simulink model "EiTR2018B (1)"  (R2019b)
settings: Solver=VariableStepAuto  StartTime=0.0  StopTime=600  RelTol=1e-3
values from neighbouring files (symbols this model uses):
  boardingTime = 15    [configFile.m]
  transportTime = 60    [configFile.m]
undefined symbols (not defined in the file or in its folder): m, n
(part 1 of 2)
settings Model: OrderedModelArguments=off  Creator=haavi  LastModifiedBy=eivin
settings DebuggingCC: ArithmeticOperatorsInVariantConditions=warning
settings SFSimCC: CustomCodeUndefinedFunction=UseInterfaceOnly

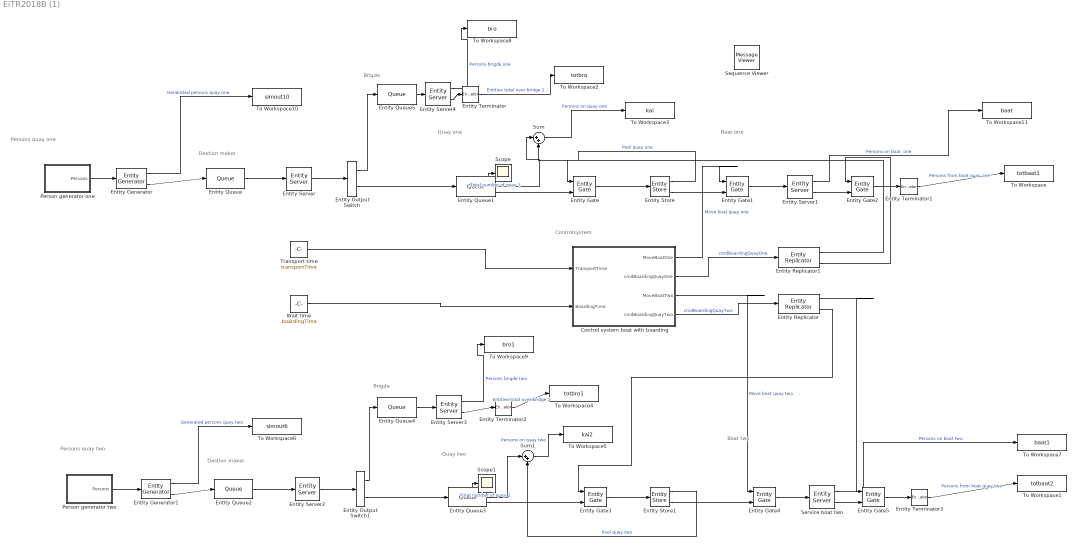
== system EiTR2018B (1) ==
  note: Controlsystem
  note: Persons quay two
  note: Boat one
  note: Quay one
  note: Brigde
  note: Destion maker
  note: Persons quay one
  note: Destion maker
  note: Brigde
  note: Quay two
  note: Boat two
  Control system boat with boarding : Stateflow chart  TreatAsAtomicUnit=on
  Entity Output Switch : EntityOutputSwitch  InputPortMessageModes=m  OutputPortMessageModes=m,m  SwitchingCriterion=From attribute  SwitchAttributeName=route
  Entity Output Switch1 : EntityOutputSwitch  InputPortMessageModes=m  OutputPortMessageModes=m,m  SwitchingCriterion=From attribute  SwitchAttributeName=route
  Entity Gate{,1..5} (6 alike) : EntityGate  InputPortMessageModes=m,m  OutputPortMessageModes=m
  Entity Generator : EntityGenerator  InputPortMessageModes=m  OutputPortMessageModes=n,m  GenerationMethod=Event-based  AttributeName=destion|route  AttributeInitialValue=-1|-1  NumberEntitiesDeparted=on  EntityType=Structured  EntityTypeName=person
      settings: InputPortMap=u0  OutputPortMap=o0,o3
  Entity Generator1 : EntityGenerator  InputPortMessageModes=m  OutputPortMessageModes=n,m  GenerationMethod=Event-based  AttributeName=destion|route  AttributeInitialValue=-1|-1  NumberEntitiesDeparted=on  EntityType=Structured  EntityTypeName=person2
      settings: InputPortMap=u0  OutputPortMap=o0,o3
  Entity Queue{,2,4..5} (4 alike) : Queue  InputPortMessageModes=m  OutputPortMessageModes=m  Capacity=inf
  Entity Queue1 : Queue  InputPortMessageModes=m  OutputPortMessageModes=n,n,m  Capacity=inf  NumberEntitiesDeparted=on  NumberEntitiesInBlock=on
      settings: OutputPortMap=o0,o1,o5
  Entity Queue3 : Queue  InputPortMessageModes=m  OutputPortMessageModes=n,n,m  Capacity=inf  NumberEntitiesDeparted=on  NumberEntitiesInBlock=on
      settings: OutputPortMap=o0,o1,o5
  Entity Replicator : EntityReplicator  InputPortMessageModes=m  OutputPortMessageModes=m,m
  Entity Replicator1 : EntityReplicator  InputPortMessageModes=m  OutputPortMessageModes=m,m
  Entity Server : EntityServer  InputPortMessageModes=m  OutputPortMessageModes=m  Capacity=inf  ServiceTimeValue=0  EntryAction=|
      | destion = 0.659;
      | entity.destion = rand();
      | 
      | if entity.destion >= destion
      |     entity.route = 1;
      | else
      |     entity.route = 2;
      | end
  Entity Server1 : EntityServer  InputPortMessageModes=m  OutputPortMessageModes=n,m  Capacity=maxPersonBoat  ServiceTimeValue=transportTime  NumberEntitiesInBlock=on
      settings: OutputPortMap=o1,o9
  Entity Server2 : EntityServer  InputPortMessageModes=m  OutputPortMessageModes=m  Capacity=inf  ServiceTimeValue=0  EntryAction=|
      | destion = 0.659;
      | entity.destion = rand();
      | 
      | if entity.destion >= destion
      |     entity.route = 1;
      | else
      |     entity.route = 2;
      | end
  Entity Server3 : EntityServer  InputPortMessageModes=m  OutputPortMessageModes=n,m  Capacity=inf  ServiceTimeValue=transportTimeBrigde  NumberEntitiesInBlock=on
      settings: OutputPortMap=o1,o9
  Entity Server4 : EntityServer  InputPortMessageModes=m  OutputPortMessageModes=n,m  Capacity=inf  ServiceTimeValue=transportTimeBrigde  NumberEntitiesInBlock=on
      settings: OutputPortMap=o1,o9
  Entity Store : EntityStore  InputPortMessageModes=m  OutputPortMessageModes=n,m  Capacity=maxPersonBoat  NumberEntitiesInBlock=on
      settings: OutputPortMap=o1,o4
  Entity Store1 : EntityStore  InputPortMessageModes=m  OutputPortMessageModes=n,m  Capacity=maxPersonBoat  NumberEntitiesInBlock=on
      settings: OutputPortMap=o1,o4
  Entity Terminator{,1..3} (4 alike) : EntityTerminator  InputPortMessageModes=m  NumberEntitiesArrived=on
      settings: OutputPortMap=o0
  Person generator one : Stateflow chart  TreatAsAtomicUnit=on
  Person generator two : Stateflow chart  TreatAsAtomicUnit=on
  Scope : Scope
  Scope1 : Scope
  Sequence Viewer : MessageViewer
  Service boat two : EntityServer  InputPortMessageModes=m  OutputPortMessageModes=n,m  Capacity=maxPersonBoat  ServiceTimeValue=transportTime  NumberEntitiesInBlock=on
      settings: OutputPortMap=o1,o9
  Sum : Sum  Inputs=|++
  Sum1 : Sum  Inputs=|++
  To Workspace : ToWorkspace  VariableName=totbaat1  SaveFormat=Timeseries  SampleTime=-1
  To Workspace1 : ToWorkspace  VariableName=totbaat2  SaveFormat=Timeseries  SampleTime=-1
  To Workspace10 : ToWorkspace  VariableName=simout10  SaveFormat=Timeseries  SampleTime=-1
  To Workspace11 : ToWorkspace  VariableName=baat  SaveFormat=Timeseries  SampleTime=-1
  To Workspace2 : ToWorkspace  VariableName=totbro  SaveFormat=Timeseries  SampleTime=-1
  To Workspace3 : ToWorkspace  VariableName=kai  SaveFormat=Timeseries  SampleTime=-1
  To Workspace4 : ToWorkspace  VariableName=totbro1  SaveFormat=Timeseries  SampleTime=-1
  To Workspace5 : ToWorkspace  VariableName=kai2  SaveFormat=Timeseries  SampleTime=-1
  To Workspace6 : ToWorkspace  VariableName=simout6  SaveFormat=Timeseries  SampleTime=-1
  To Workspace7 : ToWorkspace  VariableName=baat1  SaveFormat=Timeseries  SampleTime=-1
  To Workspace8 : ToWorkspace  VariableName=bro  SaveFormat=Timeseries  SampleTime=-1
  To Workspace9 : ToWorkspace  VariableName=bro1  SaveFormat=Timeseries  SampleTime=-1
  Transport time : Constant  Value=transportTime
  Wait time : Constant  Value=boardingTime
  wires:
  Entity Generator/2 -> Entity Queue/1
  Entity Queue/1 -> Entity Server/1
  Entity Server/1 -> Entity Output Switch/1
  Entity Output Switch/2 -> Entity Queue1/1
  Entity Generator1/2 -> Entity Queue2/1
  Entity Queue2/1 -> Entity Server2/1
  Entity Server2/1 -> Entity Output Switch1/1
  Entity Output Switch1/2 -> Entity Queue3/1
  Entity Queue3/3 -> Entity Gate3/2
  Entity Terminator1/1 -> To Workspace/1  "Persons from boat quay one"
  Entity Terminator3/1 -> To Workspace1/1  "Persons from boat quay two"
  Entity Terminator/1 -> To Workspace2/1  "Entities total over bridge 1"
  Entity Terminator2/1 -> To Workspace4/1  "Entities total over bridge 2"
  Person generator one/1(Persons) -> Entity Generator/1
  Person generator two/1(Persons) -> Entity Generator1/1
  Transport time/1 -> Control system boat with boarding/1(TransportTime)
  Wait time/1 -> Control system boat with boarding/2(BoardingTime)
  Service boat two/1 -> To Workspace7/1  "Persons on boat two"
  Entity Generator/1 -> To Workspace10/1  "Generated persons quay one"
  Entity Generator1/1 -> To Workspace6/1  "Generated persons quay two"
  Entity Queue1/3 -> Entity Gate/2
  Entity Gate/1 -> Entity Store/1
  Entity Store/2 -> Entity Gate1/2
  Control system boat with boarding/1(MoveBoatOne) -> Entity Gate1/1  "Move boat quay one"
  Entity Server1/1 -> To Workspace11/1  "Persons on boat  one"
  Entity Store/1 -> Sum/2  "Pool quay one"
  Entity Gate1/1 -> Entity Server1/1
  Entity Server1/2 -> Entity Gate2/2
  Entity Gate2/1 -> Entity Terminator1/1
  Control system boat with boarding/2(cmdBoardingQuayOne) -> Entity Replicator1/1  "cmdBoardingQuayOne"
  Entity Replicator1/1 -> Entity Gate/1
  Entity Replicator1/2 -> Entity Gate2/1
  Entity Queue1/2 -> Sum/1
  Sum/1 -> To Workspace3/1  "Persons on quay one"
  Control system boat with boarding/4(cmdBoardingQuayTwo) -> Entity Replicator/1  "cmdBoardingQuayTwo"
  Entity Gate3/1 -> Entity Store1/1
  Entity Store1/2 -> Entity Gate4/2
  Entity Gate4/1 -> Service boat two/1
  Entity Gate5/1 -> Entity Terminator3/1
  Service boat two/2 -> Entity Gate5/2
  Entity Replicator/1 -> Entity Gate5/1
  Entity Replicator/2 -> Entity Gate3/1
  Control system boat with boarding/3(MoveBoatTwo) -> Entity Gate4/1  "Move boat quay two"
  Entity Queue3/2 -> Sum1/1
  Entity Store1/1 -> Sum1/2  "Pool quay two"
  Sum1/1 -> To Workspace5/1  "Persons on quay two"
  Entity Server3/2 -> Entity Terminator2/1
  Entity Queue4/1 -> Entity Server3/1
  Entity Output Switch1/1 -> Entity Queue4/1
  Entity Output Switch/1 -> Entity Queue5/1
  Entity Queue5/1 -> Entity Server4/1
  Entity Server4/2 -> Entity Terminator/1
  Entity Server4/1 -> To Workspace8/1  "Persons brigde one"
  Entity Server3/1 -> To Workspace9/1  "Persons brigde two"
  Entity Queue1/1 -> Scope/1  "Total number of quay 1"
  Entity Queue3/1 -> Scope1/1  "Total number of quay 2"

== stateflow chart EiTR2018B (1)/Person generator one ==
  settings: enableNonTerminalStates=1
  state Hour_24
    state min_0
      state IDLE
        entry:
        lambda = 4;
        dt =60* rand();
        Persons.data=poissrnd(lambda);
      state Wait
      (default) -> Hour_24.min_0.IDLE
      Hour_24.min_0.Wait -> Hour_24.min_0.IDLE : after(dt,sec){send(Persons)}
      Hour_24.min_0.IDLE -> Hour_24.min_0.Wait
    state min_45
      state IDLE
        entry:
        lambda = 4;
        dt =60* rand();
        Persons.data=poissrnd(lambda);
      state Wait
      (default) -> Hour_24.min_45.IDLE : {dt=0;}
      Hour_24.min_45.Wait -> Hour_24.min_45.IDLE : after(dt,sec){send(Persons)}
      Hour_24.min_45.IDLE -> Hour_24.min_45.Wait
    state min_15
      state IDLE
        entry:
        lambda = 4;
        dt =60* rand();
        Persons.data=poissrnd(lambda);
      state Wait
      (default) -> Hour_24.min_15.IDLE : {dt=0;}
      Hour_24.min_15.Wait -> Hour_24.min_15.IDLE : after(dt,sec){send(Persons)}
      Hour_24.min_15.IDLE -> Hour_24.min_15.Wait
    state min_30
      state IDLE
        entry:
        lambda = 4;
        dt =60* rand();
        Persons.data=poissrnd(lambda);
      state Wait
      (default) -> Hour_24.min_30.IDLE : {dt=0;}
      Hour_24.min_30.Wait -> Hour_24.min_30.IDLE : after(dt,sec){send(Persons)}
      Hour_24.min_30.IDLE -> Hour_24.min_30.Wait
    (default) -> Hour_24.min_0
    Hour_24.min_0 -> Hour_24.min_15 : after(60*15,sec)
    Hour_24.min_30 -> Hour_24.min_45 : after(60*15,sec)
    Hour_24.min_15 -> Hour_24.min_30 : after(60*15,sec)
  state Hour_23
    state min_0
      state IDLE
        entry:
        lambda = 4;
        dt =60* rand();
        Persons.data=poissrnd(lambda);
      state Wait
      (default) -> Hour_23.min_0.IDLE
      Hour_23.min_0.Wait -> Hour_23.min_0.IDLE : after(dt,sec){send(Persons)}
      Hour_23.min_0.IDLE -> Hour_23.min_0.Wait
    state min_45
      state IDLE
        entry:
        lambda = 4;
        dt =60* rand();
        Persons.data=poissrnd(lambda);
      state Wait
      (default) -> Hour_23.min_45.IDLE : {dt=0;}
      Hour_23.min_45.Wait -> Hour_23.min_45.IDLE : after(dt,sec){send(Persons)}
      Hour_23.min_45.IDLE -> Hour_23.min_45.Wait
    state min_15
      state IDLE
        entry:
        lambda = 4;
        dt =60* rand();
        Persons.data=poissrnd(lambda);
      state Wait
      (default) -> Hour_23.min_15.IDLE : {dt=0;}
      Hour_23.min_15.Wait -> Hour_23.min_15.IDLE : after(dt,sec){send(Persons)}
      Hour_23.min_15.IDLE -> Hour_23.min_15.Wait
    state min_30
      state IDLE
        entry:
        lambda = 4;
        dt =60* rand();
        Persons.data=poissrnd(lambda);
      state Wait
      (default) -> Hour_23.min_30.IDLE : {dt=0;}
      Hour_23.min_30.Wait -> Hour_23.min_30.IDLE : after(dt,sec){send(Persons)}
      Hour_23.min_30.IDLE -> Hour_23.min_30.Wait
    (default) -> Hour_23.min_0
    Hour_23.min_0 -> Hour_23.min_15 : after(60*15,sec)
    Hour_23.min_30 -> Hour_23.min_45 : after(60*15,sec)
    Hour_23.min_15 -> Hour_23.min_30 : after(60*15,sec)
  state Hour_1
    state min_0
      state IDLE
        entry:
        lambda = 5;
        dt =60* rand()/poissrnd(lambda);
        Persons.data=poissrnd(lambda);
      state Wait
      (default) -> Hour_1.min_0.IDLE
      Hour_1.min_0.Wait -> Hour_1.min_0.IDLE : after(dt,sec){send(Persons)}
      Hour_1.min_0.IDLE -> Hour_1.min_0.Wait
    state min_45
      state IDLE
        entry:
        lambda = 4;
        dt =60* rand();
        Persons.data=poissrnd(lambda);
      state Wait
      (default) -> Hour_1.min_45.IDLE : {dt=0;}
      Hour_1.min_45.Wait -> Hour_1.min_45.IDLE : after(dt,sec){send(Persons)}
      Hour_1.min_45.IDLE -> Hour_1.min_45.Wait
    state min_15
      state IDLE
        entry:
        lambda = 40;
        dt =60* rand();
        Persons.data=poissrnd(lambda);
      state Wait
      (default) -> Hour_1.min_15.IDLE : {dt=0;}
      Hour_1.min_15.Wait -> Hour_1.min_15.IDLE : after(dt,sec){send(Persons)}
      Hour_1.min_15.IDLE -> Hour_1.min_15.Wait
    state min_30
      state IDLE
        entry:
        lambda = 4;
        dt =60* rand();
        Persons.data=poissrnd(lambda);
      state Wait
      (default) -> Hour_1.min_30.IDLE : {dt=0;}
      Hour_1.min_30.Wait -> Hour_1.min_30.IDLE : after(dt,sec){send(Persons)}
      Hour_1.min_30.IDLE -> Hour_1.min_30.Wait
    (default) -> Hour_1.min_0
    Hour_1.min_0 -> Hour_1.min_15 : after(60*15,sec)
    Hour_1.min_30 -> Hour_1.min_45 : after(60*15,sec)
    Hour_1.min_15 -> Hour_1.min_30 : after(60*15,sec)
  state Hour_22
    state min_0
      state IDLE
        entry:
        lambda = 4;
        dt =60* rand();
        Persons.data=poissrnd(lambda);
      state Wait
      (default) -> Hour_22.min_0.IDLE
      Hour_22.min_0.Wait -> Hour_22.min_0.IDLE : after(dt,sec){send(Persons)}
      Hour_22.min_0.IDLE -> Hour_22.min_0.Wait
    state min_45
      state IDLE
        entry:
        lambda = 4;
        dt =60* rand();
        Persons.data=poissrnd(lambda);
      state Wait
      (default) -> Hour_22.min_45.IDLE : {dt=0;}
      Hour_22.min_45.Wait -> Hour_22.min_45.IDLE : after(dt,sec){send(Persons)}
      Hour_22.min_45.IDLE -> Hour_22.min_45.Wait
    state min_15
      state IDLE
        entry:
        lambda = 4;
        dt =60* rand();
        Persons.data=poissrnd(lambda);
      state Wait
      (default) -> Hour_22.min_15.IDLE : {dt=0;}
      Hour_22.min_15.Wait -> Hour_22.min_15.IDLE : after(dt,sec){send(Persons)}
      Hour_22.min_15.IDLE -> Hour_22.min_15.Wait
    state min_30
      state IDLE
        entry:
        lambda = 4;
        dt =60* rand();
        Persons.data=poissrnd(lambda);
      state Wait
      (default) -> Hour_22.min_30.IDLE : {dt=0;}
      Hour_22.min_30.Wait -> Hour_22.min_30.IDLE : after(dt,sec){send(Persons)}
      Hour_22.min_30.IDLE -> Hour_22.min_30.Wait
    (default) -> Hour_22.min_0
    Hour_22.min_0 -> Hour_22.min_15 : after(60*15,sec)
    Hour_22.min_30 -> Hour_22.min_45 : after(60*15,sec)
    Hour_22.min_15 -> Hour_22.min_30 : after(60*15,sec)
  state Hour_2
    state min_0
      state IDLE
        entry:
        lambda = 4;
        dt =60* rand();
        Persons.data=poissrnd(lambda);
      state Wait
      (default) -> Hour_2.min_0.IDLE
      Hour_2.min_0.Wait -> Hour_2.min_0.IDLE : after(dt,sec){send(Persons)}
      Hour_2.min_0.IDLE -> Hour_2.min_0.Wait
    state min_45
      state IDLE
        entry:
        lambda = 4;
        dt =60* rand();
        Persons.data=poissrnd(lambda);
      state Wait
      (default) -> Hour_2.min_45.IDLE : {dt=0;}
      Hour_2.min_45.Wait -> Hour_2.min_45.IDLE : after(dt,sec){send(Persons)}
      Hour_2.min_45.IDLE -> Hour_2.min_45.Wait
    state min_15
      state IDLE
        entry:
        lambda = 4;
        dt =60* rand();
        Persons.data=poissrnd(lambda);
      state Wait
      (default) -> Hour_2.min_15.IDLE : {dt=0;}
      Hour_2.min_15.Wait -> Hour_2.min_15.IDLE : after(dt,sec){send(Persons)}
      Hour_2.min_15.IDLE -> Hour_2.min_15.Wait
    state min_30
      state IDLE
        entry:
        lambda = 4;
        dt =60* rand();
        Persons.data=poissrnd(lambda);
      state Wait
      (default) -> Hour_2.min_30.IDLE : {dt=0;}
      Hour_2.min_30.Wait -> Hour_2.min_30.IDLE : after(dt,sec){send(Persons)}
      Hour_2.min_30.IDLE -> Hour_2.min_30.Wait
    (default) -> Hour_2.min_0
    Hour_2.min_0 -> Hour_2.min_15 : after(60*15,sec)
    Hour_2.min_30 -> Hour_2.min_45 : after(60*15,sec)
    Hour_2.min_15 -> Hour_2.min_30 : after(60*15,sec)
  state Hour_21
    state min_0
      state IDLE
        entry:
        lambda = 4;
        dt =60* rand();
        Persons.data=poissrnd(lambda);
      state Wait
      (default) -> Hour_21.min_0.IDLE
      Hour_21.min_0.Wait -> Hour_21.min_0.IDLE : after(dt,sec){send(Persons)}
      Hour_21.min_0.IDLE -> Hour_21.min_0.Wait
    state min_45
      state IDLE
        entry:
        lambda = 4;
        dt =60* rand();
        Persons.data=poissrnd(lambda);
      state Wait
      (default) -> Hour_21.min_45.IDLE : {dt=0;}
      Hour_21.min_45.Wait -> Hour_21.min_45.IDLE : after(dt,sec){send(Persons)}
      Hour_21.min_45.IDLE -> Hour_21.min_45.Wait
    state min_15
      state IDLE
        entry:
        lambda = 4;
        dt =60* rand();
        Persons.data=poissrnd(lambda);
      state Wait
      (default) -> Hour_21.min_15.IDLE : {dt=0;}
      Hour_21.min_15.Wait -> Hour_21.min_15.IDLE : after(dt,sec){send(Persons)}
      Hour_21.min_15.IDLE -> Hour_21.min_15.Wait
    state min_30
      state IDLE
        entry:
        lambda = 4;
        dt =60* rand();
        Persons.data=poissrnd(lambda);
      state Wait
      (default) -> Hour_21.min_30.IDLE : {dt=0;}
      Hour_21.min_30.Wait -> Hour_21.min_30.IDLE : after(dt,sec){send(Persons)}
      Hour_21.min_30.IDLE -> Hour_21.min_30.Wait
    (default) -> Hour_21.min_0
    Hour_21.min_0 -> Hour_21.min_15 : after(60*15,sec)
    Hour_21.min_30 -> Hour_21.min_45 : after(60*15,sec)
    Hour_21.min_15 -> Hour_21.min_30 : after(60*15,sec)
  state Hour_3
    state min_0
      state IDLE
        entry:
        lambda = 4;
        dt =60* rand();
        Persons.data=poissrnd(lambda);
      state Wait
      (default) -> Hour_3.min_0.IDLE
      Hour_3.min_0.Wait -> Hour_3.min_0.IDLE : after(dt,sec){send(Persons)}
      Hour_3.min_0.IDLE -> Hour_3.min_0.Wait
    state min_45
      state IDLE
        entry:
        lambda = 4;
        dt =60* rand();
        Persons.data=poissrnd(lambda);
      state Wait
      (default) -> Hour_3.min_45.IDLE : {dt=0;}
      Hour_3.min_45.Wait -> Hour_3.min_45.IDLE : after(dt,sec){send(Persons)}
      Hour_3.min_45.IDLE -> Hour_3.min_45.Wait
    state min_15
      state IDLE
        entry:
        lambda = 4;
        dt =60* rand();
        Persons.data=poissrnd(lambda);
      state Wait
      (default) -> Hour_3.min_15.IDLE : {dt=0;}
      Hour_3.min_15.Wait -> Hour_3.min_15.IDLE : after(dt,sec){send(Persons)}
      Hour_3.min_15.IDLE -> Hour_3.min_15.Wait
    state min_30
      state IDLE
        entry:
        lambda = 4;
        dt =60* rand();
        Persons.data=poissrnd(lambda);
      state Wait
      (default) -> Hour_3.min_30.IDLE : {dt=0;}
      Hour_3.min_30.Wait -> Hour_3.min_30.IDLE : after(dt,sec){send(Persons)}
      Hour_3.min_30.IDLE -> Hour_3.min_30.Wait
    (default) -> Hour_3.min_0
    Hour_3.min_0 -> Hour_3.min_15 : after(60*15,sec)
    Hour_3.min_30 -> Hour_3.min_45 : after(60*15,sec)
    Hour_3.min_15 -> Hour_3.min_30 : after(60*15,sec)
  state Hour_20
    state min_0
      state IDLE
        entry:
        lambda = 4;
        dt =60* rand();
        Persons.data=poissrnd(lambda);
      state Wait
      (default) -> Hour_20.min_0.IDLE
      Hour_20.min_0.Wait -> Hour_20.min_0.IDLE : after(dt,sec){send(Persons)}
      Hour_20.min_0.IDLE -> Hour_20.min_0.Wait
    state min_45
      state IDLE
        entry:
        lambda = 4;
        dt =60* rand();
        Persons.data=poissrnd(lambda);
      state Wait
      (default) -> Hour_20.min_45.IDLE : {dt=0;}
      Hour_20.min_45.Wait -> Hour_20.min_45.IDLE : after(dt,sec){send(Persons)}
      Hour_20.min_45.IDLE -> Hour_20.min_45.Wait
    state min_15
      state IDLE
        entry:
        lambda = 4;
        dt =60* rand();
        Persons.data=poissrnd(lambda);
      state Wait
      (default) -> Hour_20.min_15.IDLE : {dt=0;}
      Hour_20.min_15.Wait -> Hour_20.min_15.IDLE : after(dt,sec){send(Persons)}
      Hour_20.min_15.IDLE -> Hour_20.min_15.Wait
    state min_30
      state IDLE
        entry:
        lambda = 4;
        dt =60* rand();
        Persons.data=poissrnd(lambda);
      state Wait
      (default) -> Hour_20.min_30.IDLE : {dt=0;}
      Hour_20.min_30.Wait -> Hour_20.min_30.IDLE : after(dt,sec){send(Persons)}
      Hour_20.min_30.IDLE -> Hour_20.min_30.Wait
    (default) -> Hour_20.min_0
    Hour_20.min_0 -> Hour_20.min_15 : after(60*15,sec)
    Hour_20.min_30 -> Hour_20.min_45 : after(60*15,sec)
    Hour_20.min_15 -> Hour_20.min_30 : after(60*15,sec)
  state Hour_4
    state min_0
      state IDLE
        entry:
        lambda = 4;
        dt =60* rand();
        Persons.data=poissrnd(lambda);
      state Wait
      (default) -> Hour_4.min_0.IDLE
      Hour_4.min_0.Wait -> Hour_4.min_0.IDLE : after(dt,sec){send(Persons)}
      Hour_4.min_0.IDLE -> Hour_4.min_0.Wait
    state min_45
      state IDLE
        entry:
        lambda = 4;
        dt =60* rand();
        Persons.data=poissrnd(lambda);
      state Wait
      (default) -> Hour_4.min_45.IDLE : {dt=0;}
      Hour_4.min_45.Wait -> Hour_4.min_45.IDLE : after(dt,sec){send(Persons)}
      Hour_4.min_45.IDLE -> Hour_4.min_45.Wait
    state min_15
      state IDLE
        entry:
        lambda = 4;
        dt =60* rand();
        Persons.data=poissrnd(lambda);
      state Wait
      (default) -> Hour_4.min_15.IDLE : {dt=0;}
      Hour_4.min_15.Wait -> Hour_4.min_15.IDLE : after(dt,sec){send(Persons)}
      Hour_4.min_15.IDLE -> Hour_4.min_15.Wait
    state min_30
      state IDLE
        entry:
        lambda = 4;
        dt =60* rand();
        Persons.data=poissrnd(lambda);
      state Wait
      (default) -> Hour_4.min_30.IDLE : {dt=0;}
      Hour_4.min_30.Wait -> Hour_4.min_30.IDLE : after(dt,sec){send(Persons)}
      Hour_4.min_30.IDLE -> Hour_4.min_30.Wait
    (default) -> Hour_4.min_0
    Hour_4.min_0 -> Hour_4.min_15 : after(60*15,sec)
    Hour_4.min_30 -> Hour_4.min_45 : after(60*15,sec)
    Hour_4.min_15 -> Hour_4.min_30 : after(60*15,sec)
  state Hour_19
    state min_0
      state IDLE
        entry:
        lambda = 4;
        dt =60* rand();
        Persons.data=poissrnd(lambda);
      state Wait
      (default) -> Hour_19.min_0.IDLE
      Hour_19.min_0.Wait -> Hour_19.min_0.IDLE : after(dt,sec){send(Persons)}
      Hour_19.min_0.IDLE -> Hour_19.min_0.Wait
    state min_45
      state IDLE
        entry:
        lambda = 4;
        dt =60* rand();
        Persons.data=poissrnd(lambda);
      state Wait
      (default) -> Hour_19.min_45.IDLE : {dt=0;}
      Hour_19.min_45.Wait -> Hour_19.min_45.IDLE : after(dt,sec){send(Persons)}
      Hour_19.min_45.IDLE -> Hour_19.min_45.Wait
    state min_15
      state IDLE
        entry:
        lambda = 4;
        dt =60* rand();
        Persons.data=poissrnd(lambda);
      state Wait
      (default) -> Hour_19.min_15.IDLE : {dt=0;}
      Hour_19.min_15.Wait -> Hour_19.min_15.IDLE : after(dt,sec){send(Persons)}
      Hour_19.min_15.IDLE -> Hour_19.min_15.Wait
    state min_30
      state IDLE
        entry:
        lambda = 4;
        dt =60* rand();
        Persons.data=poissrnd(lambda);
      state Wait
      (default) -> Hour_19.min_30.IDLE : {dt=0;}
      Hour_19.min_30.Wait -> Hour_19.min_30.IDLE : after(dt,sec){send(Persons)}
      Hour_19.min_30.IDLE -> Hour_19.min_30.Wait
    (default) -> Hour_19.min_0
    Hour_19.min_0 -> Hour_19.min_15 : after(60*15,sec)
    Hour_19.min_30 -> Hour_19.min_45 : after(60*15,sec)
    Hour_19.min_15 -> Hour_19.min_30 : after(60*15,sec)
  state Hour_5
    state min_0
      state IDLE
        entry:
        lambda = 4;
        dt =60* rand();
        Persons.data=poissrnd(lambda);
      state Wait
      (default) -> Hour_5.min_0.IDLE
      Hour_5.min_0.Wait -> Hour_5.min_0.IDLE : after(dt,sec){send(Persons)}
      Hour_5.min_0.IDLE -> Hour_5.min_0.Wait
    state min_45
      state IDLE
        entry:
        lambda = 4;
        dt =60* rand();
        Persons.data=poissrnd(lambda);
      state Wait
      (default) -> Hour_5.min_45.IDLE : {dt=0;}
      Hour_5.min_45.Wait -> Hour_5.min_45.IDLE : after(dt,sec){send(Persons)}
      Hour_5.min_45.IDLE -> Hour_5.min_45.Wait
    state min_15
      state IDLE
        entry:
        lambda = 4;
        dt =60* rand();
        Persons.data=poissrnd(lambda);
      state Wait
      (default) -> Hour_5.min_15.IDLE : {dt=0;}
      Hour_5.min_15.Wait -> Hour_5.min_15.IDLE : after(dt,sec){send(Persons)}
      Hour_5.min_15.IDLE -> Hour_5.min_15.Wait
    state min_30
      state IDLE
        entry:
        lambda = 4;
        dt =60* rand();
        Persons.data=poissrnd(lambda);
      state Wait
      (default) -> Hour_5.min_30.IDLE : {dt=0;}
      Hour_5.min_30.Wait -> Hour_5.min_30.IDLE : after(dt,sec){send(Persons)}
      Hour_5.min_30.IDLE -> Hour_5.min_30.Wait
    (default) -> Hour_5.min_0
    Hour_5.min_0 -> Hour_5.min_15 : after(60*15,sec)
    Hour_5.min_30 -> Hour_5.min_45 : after(60*15,sec)
    Hour_5.min_15 -> Hour_5.min_30 : after(60*15,sec)
  state Hour_18
    state min_0
      state IDLE
        entry:
        lambda = 4;
        dt =60* rand();
        Persons.data=poissrnd(lambda);
      state Wait
      (default) -> Hour_18.min_0.IDLE
      Hour_18.min_0.Wait -> Hour_18.min_0.IDLE : after(dt,sec){send(Persons)}
      Hour_18.min_0.IDLE -> Hour_18.min_0.Wait
    state min_45
      state IDLE
        entry:
        lambda = 4;
        dt =60* rand();
        Persons.data=poissrnd(lambda);
      state Wait
      (default) -> Hour_18.min_45.IDLE : {dt=0;}
      Hour_18.min_45.Wait -> Hour_18.min_45.IDLE : after(dt,sec){send(Persons)}
      Hour_18.min_45.IDLE -> Hour_18.min_45.Wait
    state min_15
      state IDLE
        entry:
        lambda = 4;
        dt =60* rand();
        Persons.data=poissrnd(lambda);
      state Wait
      (default) -> Hour_18.min_15.IDLE : {dt=0;}
      Hour_18.min_15.Wait -> Hour_18.min_15.IDLE : after(dt,sec){send(Persons)}
      Hour_18.min_15.IDLE -> Hour_18.min_15.Wait
    state min_30
      state IDLE
        entry:
        lambda = 4;
        dt =60* rand();
        Persons.data=poissrnd(lambda);
      state Wait
      (default) -> Hour_18.min_30.IDLE : {dt=0;}
      Hour_18.min_30.Wait -> Hour_18.min_30.IDLE : after(dt,sec){send(Persons)}
      Hour_18.min_30.IDLE -> Hour_18.min_30.Wait
    (default) -> Hour_18.min_0
    Hour_18.min_0 -> Hour_18.min_15 : after(60*15,sec)
    Hour_18.min_30 -> Hour_18.min_45 : after(60*15,sec)
    Hour_18.min_15 -> Hour_18.min_30 : after(60*15,sec)
  state Hour_6
    state min_0
      state IDLE
        entry:
        lambda = 4;
        dt =60* rand();
        Persons.data=poissrnd(lambda);
      state Wait
      (default) -> Hour_6.min_0.IDLE
      Hour_6.min_0.Wait -> Hour_6.min_0.IDLE : after(dt,sec){send(Persons)}
      Hour_6.min_0.IDLE -> Hour_6.min_0.Wait
    state min_45
      state IDLE
        entry:
        lambda = 4;
        dt =60* rand();
        Persons.data=poissrnd(lambda);
      state Wait
      (default) -> Hour_6.min_45.IDLE : {dt=0;}
      Hour_6.min_45.Wait -> Hour_6.min_45.IDLE : after(dt,sec){send(Persons)}
      Hour_6.min_45.IDLE -> Hour_6.min_45.Wait
    state min_15
      state IDLE
        entry:
        lambda = 4;
        dt =60* rand();
        Persons.data=poissrnd(lambda);
      state Wait
      (default) -> Hour_6.min_15.IDLE : {dt=0;}
      Hour_6.min_15.Wait -> Hour_6.min_15.IDLE : after(dt,sec){send(Persons)}
      Hour_6.min_15.IDLE -> Hour_6.min_15.Wait
    state min_30
      state IDLE
        entry:
        lambda = 4;
        dt =60* rand();
        Persons.data=poissrnd(lambda);
      state Wait
      (default) -> Hour_6.min_30.IDLE : {dt=0;}
      Hour_6.min_30.Wait -> Hour_6.min_30.IDLE : after(dt,sec){send(Persons)}
      Hour_6.min_30.IDLE -> Hour_6.min_30.Wait
    (default) -> Hour_6.min_0
    Hour_6.min_0 -> Hour_6.min_15 : after(60*15,sec)
    Hour_6.min_30 -> Hour_6.min_45 : after(60*15,sec)
    Hour_6.min_15 -> Hour_6.min_30 : after(60*15,sec)
  state Hour_17
    state min_0
      state IDLE
        entry:
        lambda = 4;
        dt =60* rand();
        Persons.data=poissrnd(lambda);
      state Wait
      (default) -> Hour_17.min_0.IDLE
      Hour_17.min_0.Wait -> Hour_17.min_0.IDLE : after(dt,sec){send(Persons)}
      Hour_17.min_0.IDLE -> Hour_17.min_0.Wait
    state min_45
      state IDLE
        entry:
        lambda = 4;
        dt =60* rand();
        Persons.data=poissrnd(lambda);
      state Wait
      (default) -> Hour_17.min_45.IDLE : {dt=0;}
      Hour_17.min_45.Wait -> Hour_17.min_45.IDLE : after(dt,sec){send(Persons)}
      Hour_17.min_45.IDLE -> Hour_17.min_45.Wait
    state min_15
      state IDLE
        entry:
        lambda = 4;
        dt =60* rand();
        Persons.data=poissrnd(lambda);
      state Wait
      (default) -> Hour_17.min_15.IDLE : {dt=0;}
      Hour_17.min_15.Wait -> Hour_17.min_15.IDLE : after(dt,sec){send(Persons)}
      Hour_17.min_15.IDLE -> Hour_17.min_15.Wait
    state min_30
      state IDLE
        entry:
        lambda = 4;
        dt =60* rand();
        Persons.data=poissrnd(lambda);
      state Wait
      (default) -> Hour_17.min_30.IDLE : {dt=0;}
      Hour_17.min_30.Wait -> Hour_17.min_30.IDLE : after(dt,sec){send(Persons)}
      Hour_17.min_30.IDLE -> Hour_17.min_30.Wait
    (default) -> Hour_17.min_0
    Hour_17.min_0 -> Hour_17.min_15 : after(60*15,sec)
    Hour_17.min_30 -> Hour_17.min_45 : after(60*15,sec)
    Hour_17.min_15 -> Hour_17.min_30 : after(60*15,sec)
  state Hour_7
    state min_0
      state IDLE
        entry:
        lambda = 4;
        dt =60* rand();
        Persons.data=poissrnd(lambda);
      state Wait
      (default) -> Hour_7.min_0.IDLE
      Hour_7.min_0.Wait -> Hour_7.min_0.IDLE : after(dt,sec){send(Persons)}
      Hour_7.min_0.IDLE -> Hour_7.min_0.Wait
    state min_45
      state IDLE
        entry:
        lambda = 4;
        dt =60* rand();
        Persons.data=poissrnd(lambda);
      state Wait
      (default) -> Hour_7.min_45.IDLE : {dt=0;}
      Hour_7.min_45.Wait -> Hour_7.min_45.IDLE : after(dt,sec){send(Persons)}
      Hour_7.min_45.IDLE -> Hour_7.min_45.Wait
    state min_15
      state IDLE
        entry:
        lambda = 4;
        dt =60* rand();
        Persons.data=poissrnd(lambda);
      state Wait
      (default) -> Hour_7.min_15.IDLE : {dt=0;}
      Hour_7.min_15.Wait -> Hour_7.min_15.IDLE : after(dt,sec){send(Persons)}
      Hour_7.min_15.IDLE -> Hour_7.min_15.Wait
    state min_30
      state IDLE
        entry:
        lambda = 4;
        dt =60* rand();
        Persons.data=poissrnd(lambda);
      state Wait
      (default) -> Hour_7.min_30.IDLE : {dt=0;}
      Hour_7.min_30.Wait -> Hour_7.min_30.IDLE : after(dt,sec){send(Persons)}
      Hour_7.min_30.IDLE -> Hour_7.min_30.Wait
    (default) -> Hour_7.min_0
    Hour_7.min_0 -> Hour_7.min_15 : after(60*15,sec)
    Hour_7.min_30 -> Hour_7.min_45 : after(60*15,sec)
    Hour_7.min_15 -> Hour_7.min_30 : after(60*15,sec)
  state Hour_16
    state min_0
      state IDLE
        entry:
        lambda = 4;
        dt =60* rand();
        Persons.data=poissrnd(lambda);
      state Wait
      (default) -> Hour_16.min_0.IDLE
      Hour_16.min_0.Wait -> Hour_16.min_0.IDLE : after(dt,sec){send(Persons)}
      Hour_16.min_0.IDLE -> Hour_16.min_0.Wait
    state min_45
      state IDLE
        entry:
        lambda = 4;
        dt =60* rand();
        Persons.data=poissrnd(lambda);
      state Wait
      (default) -> Hour_16.min_45.IDLE : {dt=0;}
      Hour_16.min_45.Wait -> Hour_16.min_45.IDLE : after(dt,sec){send(Persons)}
      Hour_16.min_45.IDLE -> Hour_16.min_45.Wait
    state min_15
      state IDLE
        entry:
        lambda = 4;
        dt =60* rand();
        Persons.data=poissrnd(lambda);
      state Wait
      (default) -> Hour_16.min_15.IDLE : {dt=0;}
      Hour_16.min_15.Wait -> Hour_16.min_15.IDLE : after(dt,sec){send(Persons)}
      Hour_16.min_15.IDLE -> Hour_16.min_15.Wait
    state min_30
      state IDLE
        entry:
        lambda = 4;
        dt =60* rand();
        Persons.data=poissrnd(lambda);
      state Wait
      (default) -> Hour_16.min_30.IDLE : {dt=0;}
      Hour_16.min_30.Wait -> Hour_16.min_30.IDLE : after(dt,sec){send(Persons)}
      Hour_16.min_30.IDLE -> Hour_16.min_30.Wait
    (default) -> Hour_16.min_0
    Hour_16.min_0 -> Hour_16.min_15 : after(60*15,sec)
    Hour_16.min_30 -> Hour_16.min_45 : after(60*15,sec)
    Hour_16.min_15 -> Hour_16.min_30 : after(60*15,sec)
  state Hour_8
    state min_0
      state IDLE
        entry:
        lambda = 4;
        dt =60* rand();
        Persons.data=poissrnd(lambda);
      state Wait
      (default) -> Hour_8.min_0.IDLE
      Hour_8.min_0.Wait -> Hour_8.min_0.IDLE : after(dt,sec){send(Persons)}
      Hour_8.min_0.IDLE -> Hour_8.min_0.Wait
    state min_45
      state IDLE
        entry:
        lambda = 4;
        dt =60* rand();
        Persons.data=poissrnd(lambda);
      state Wait
      (default) -> Hour_8.min_45.IDLE : {dt=0;}
      Hour_8.min_45.Wait -> Hour_8.min_45.IDLE : after(dt,sec){send(Persons)}
      Hour_8.min_45.IDLE -> Hour_8.min_45.Wait
    state min_15
      state IDLE
        entry:
        lambda = 4;
        dt =60* rand();
        Persons.data=poissrnd(lambda);
      state Wait
      (default) -> Hour_8.min_15.IDLE : {dt=0;}
      Hour_8.min_15.Wait -> Hour_8.min_15.IDLE : after(dt,sec){send(Persons)}
      Hour_8.min_15.IDLE -> Hour_8.min_15.Wait
    state min_30
      state IDLE
        entry:
        lambda = 4;
        dt =60* rand();
        Persons.data=poissrnd(lambda);
      state Wait
      (default) -> Hour_8.min_30.IDLE : {dt=0;}
      Hour_8.min_30.Wait -> Hour_8.min_30.IDLE : after(dt,sec){send(Persons)}
      Hour_8.min_30.IDLE -> Hour_8.min_30.Wait
    (default) -> Hour_8.min_0
    Hour_8.min_0 -> Hour_8.min_15 : after(60*15,sec)
    Hour_8.min_30 -> Hour_8.min_45 : after(60*15,sec)
    Hour_8.min_15 -> Hour_8.min_30 : after(60*15,sec)
  state Hour_15
    state min_0
      state IDLE
        entry:
        lambda = 4;
        dt =60* rand();
        Persons.data=poissrnd(lambda);
      state Wait
      (default) -> Hour_15.min_0.IDLE
      Hour_15.min_0.Wait -> Hour_15.min_0.IDLE : after(dt,sec){send(Persons)}
      Hour_15.min_0.IDLE -> Hour_15.min_0.Wait
    state min_45
      state IDLE
        entry:
        lambda = 4;
        dt =60* rand();
        Persons.data=poissrnd(lambda);
      state Wait
      (default) -> Hour_15.min_45.IDLE : {dt=0;}
      Hour_15.min_45.Wait -> Hour_15.min_45.IDLE : after(dt,sec){send(Persons)}
      Hour_15.min_45.IDLE -> Hour_15.min_45.Wait
    state min_15
      state IDLE
        entry:
        lambda = 4;
        dt =60* rand();
        Persons.data=poissrnd(lambda);
      state Wait
      (default) -> Hour_15.min_15.IDLE : {dt=0;}
      Hour_15.min_15.Wait -> Hour_15.min_15.IDLE : after(dt,sec){send(Persons)}
      Hour_15.min_15.IDLE -> Hour_15.min_15.Wait
    state min_30
      state IDLE
        entry:
        lambda = 4;
        dt =60* rand();
        Persons.data=poissrnd(lambda);
      state Wait
      (default) -> Hour_15.min_30.IDLE : {dt=0;}
      Hour_15.min_30.Wait -> Hour_15.min_30.IDLE : after(dt,sec){send(Persons)}
      Hour_15.min_30.IDLE -> Hour_15.min_30.Wait
    (default) -> Hour_15.min_0
    Hour_15.min_0 -> Hour_15.min_15 : after(60*15,sec)
    Hour_15.min_30 -> Hour_15.min_45 : after(60*15,sec)
    Hour_15.min_15 -> Hour_15.min_30 : after(60*15,sec)
  state Hour_14
    state min_0
      state IDLE
        entry:
        lambda = 4;
        dt =60* rand();
        Persons.data=poissrnd(lambda);
      state Wait
      (default) -> Hour_14.min_0.IDLE
      Hour_14.min_0.Wait -> Hour_14.min_0.IDLE : after(dt,sec){send(Persons)}
      Hour_14.min_0.IDLE -> Hour_14.min_0.Wait
    state min_45
      state IDLE
        entry:
        lambda = 4;
        dt =60* rand();
        Persons.data=poissrnd(lambda);
      state Wait
      (default) -> Hour_14.min_45.IDLE : {dt=0;}
      Hour_14.min_45.Wait -> Hour_14.min_45.IDLE : after(dt,sec){send(Persons)}
      Hour_14.min_45.IDLE -> Hour_14.min_45.Wait
    state min_15
      state IDLE
        entry:
        lambda = 4;
        dt =60* rand();
        Persons.data=poissrnd(lambda);
      state Wait
      (default) -> Hour_14.min_15.IDLE : {dt=0;}
      Hour_14.min_15.Wait -> Hour_14.min_15.IDLE : after(dt,sec){send(Persons)}
      Hour_14.min_15.IDLE -> Hour_14.min_15.Wait
    state min_30
      state IDLE
        entry:
        lambda = 4;
        dt =60* rand();
        Persons.data=poissrnd(lambda);
      state Wait
      (default) -> Hour_14.min_30.IDLE : {dt=0;}
      Hour_14.min_30.Wait -> Hour_14.min_30.IDLE : after(dt,sec){send(Persons)}
      Hour_14.min_30.IDLE -> Hour_14.min_30.Wait
    (default) -> Hour_14.min_0
    Hour_14.min_0 -> Hour_14.min_15 : after(60*15,sec)
    Hour_14.min_30 -> Hour_14.min_45 : after(60*15,sec)
    Hour_14.min_15 -> Hour_14.min_30 : after(60*15,sec)
  state Hour_9
    state min_0
      state IDLE
        entry:
        lambda = 4;
        dt =60* rand();
        Persons.data=poissrnd(lambda);
      state Wait
      (default) -> Hour_9.min_0.IDLE
      Hour_9.min_0.Wait -> Hour_9.min_0.IDLE : after(dt,sec){send(Persons)}
      Hour_9.min_0.IDLE -> Hour_9.min_0.Wait
    state min_45
      state IDLE
        entry:
        lambda = 4;
        dt =60* rand();
        Persons.data=poissrnd(lambda);
      state Wait
      (default) -> Hour_9.min_45.IDLE : {dt=0;}
      Hour_9.min_45.Wait -> Hour_9.min_45.IDLE : after(dt,sec){send(Persons)}
      Hour_9.min_45.IDLE -> Hour_9.min_45.Wait
    state min_15
      state IDLE
        entry:
        lambda = 4;
        dt =60* rand();
        Persons.data=poissrnd(lambda);
      state Wait
      (default) -> Hour_9.min_15.IDLE : {dt=0;}
      Hour_9.min_15.Wait -> Hour_9.min_15.IDLE : after(dt,sec){send(Persons)}
      Hour_9.min_15.IDLE -> Hour_9.min_15.Wait
    state min_30
      state IDLE
        entry:
        lambda = 4;
        dt =60* rand();
        Persons.data=poissrnd(lambda);
      state Wait
      (default) -> Hour_9.min_30.IDLE : {dt=0;}
      Hour_9.min_30.Wait -> Hour_9.min_30.IDLE : after(dt,sec){send(Persons)}
      Hour_9.min_30.IDLE -> Hour_9.min_30.Wait
    (default) -> Hour_9.min_0
    Hour_9.min_0 -> Hour_9.min_15 : after(60*15,sec)
    Hour_9.min_30 -> Hour_9.min_45 : after(60*15,sec)
    Hour_9.min_15 -> Hour_9.min_30 : after(60*15,sec)
  state Hour_10
    state min_0
      state IDLE
        entry:
        lambda = 4;
        dt =60* rand();
        Persons.data=poissrnd(lambda);
      state Wait
      (default) -> Hour_10.min_0.IDLE
      Hour_10.min_0.Wait -> Hour_10.min_0.IDLE : after(dt,sec){send(Persons)}
      Hour_10.min_0.IDLE -> Hour_10.min_0.Wait
    state min_45
      state IDLE
        entry:
        lambda = 4;
        dt =60* rand();
        Persons.data=poissrnd(lambda);
      state Wait
      (default) -> Hour_10.min_45.IDLE : {dt=0;}
      Hour_10.min_45.Wait -> Hour_10.min_45.IDLE : after(dt,sec){send(Persons)}
      Hour_10.min_45.IDLE -> Hour_10.min_45.Wait
    state min_15
      state IDLE
        entry:
        lambda = 4;
        dt =60* rand();
        Persons.data=poissrnd(lambda);
      state Wait
      (default) -> Hour_10.min_15.IDLE : {dt=0;}
      Hour_10.min_15.Wait -> Hour_10.min_15.IDLE : after(dt,sec){send(Persons)}
      Hour_10.min_15.IDLE -> Hour_10.min_15.Wait
    state min_30
      state IDLE
        entry:
        lambda = 4;
        dt =60* rand();
        Persons.data=poissrnd(lambda);
      state Wait
      (default) -> Hour_10.min_30.IDLE : {dt=0;}
      Hour_10.min_30.Wait -> Hour_10.min_30.IDLE : after(dt,sec){send(Persons)}
      Hour_10.min_30.IDLE -> Hour_10.min_30.Wait
    (default) -> Hour_10.min_0
    Hour_10.min_0 -> Hour_10.min_15 : after(60*15,sec)
    Hour_10.min_30 -> Hour_10.min_45 : after(60*15,sec)
    Hour_10.min_15 -> Hour_10.min_30 : after(60*15,sec)
  state Hour_13
    state min_0
      state IDLE
        entry:
        lambda = 4;
        dt =60* rand();
        Persons.data=poissrnd(lambda);
      state Wait
      (default) -> Hour_13.min_0.IDLE
      Hour_13.min_0.Wait -> Hour_13.min_0.IDLE : after(dt,sec){send(Persons)}
      Hour_13.min_0.IDLE -> Hour_13.min_0.Wait
    state min_45
      state IDLE
        entry:
        lambda = 4;
        dt =60* rand();
        Persons.data=poissrnd(lambda);
      state Wait
      (default) -> Hour_13.min_45.IDLE : {dt=0;}
      Hour_13.min_45.Wait -> Hour_13.min_45.IDLE : after(dt,sec){send(Persons)}
      Hour_13.min_45.IDLE -> Hour_13.min_45.Wait
    state min_15
      state IDLE
        entry:
        lambda = 4;
        dt =60* rand();
        Persons.data=poissrnd(lambda);
      state Wait
      (default) -> Hour_13.min_15.IDLE : {dt=0;}
      Hour_13.min_15.Wait -> Hour_13.min_15.IDLE : after(dt,sec){send(Persons)}
      Hour_13.min_15.IDLE -> Hour_13.min_15.Wait
    state min_30
      state IDLE
        entry:
        lambda = 4;
        dt =60* rand();
        Persons.data=poissrnd(lambda);
      state Wait
      (default) -> Hour_13.min_30.IDLE : {dt=0;}
      Hour_13.min_30.Wait -> Hour_13.min_30.IDLE : after(dt,sec){send(Persons)}
      Hour_13.min_30.IDLE -> Hour_13.min_30.Wait
    (default) -> Hour_13.min_0
    Hour_13.min_0 -> Hour_13.min_15 : after(60*15,sec)
    Hour_13.min_30 -> Hour_13.min_45 : after(60*15,sec)
    Hour_13.min_15 -> Hour_13.min_30 : after(60*15,sec)
  state Hour_11
    state min_0
      state IDLE
        entry:
        lambda = 4;
        dt =60* rand();
        Persons.data=poissrnd(lambda);
      state Wait
      (default) -> Hour_11.min_0.IDLE
      Hour_11.min_0.Wait -> Hour_11.min_0.IDLE : after(dt,sec){send(Persons)}
      Hour_11.min_0.IDLE -> Hour_11.min_0.Wait
    state min_45
      state IDLE
        entry:
        lambda = 4;
        dt =60* rand();
        Persons.data=poissrnd(lambda);
      state Wait
      (default) -> Hour_11.min_45.IDLE : {dt=0;}
      Hour_11.min_45.Wait -> Hour_11.min_45.IDLE : after(dt,sec){send(Persons)}
      Hour_11.min_45.IDLE -> Hour_11.min_45.Wait
    state min_15
      state IDLE
        entry:
        lambda = 4;
        dt =60* rand();
        Persons.data=poissrnd(lambda);
      state Wait
      (default) -> Hour_11.min_15.IDLE : {dt=0;}
      Hour_11.min_15.Wait -> Hour_11.min_15.IDLE : after(dt,sec){send(Persons)}
      Hour_11.min_15.IDLE -> Hour_11.min_15.Wait
    state min_30
      state IDLE
        entry:
        lambda = 4;
        dt =60* rand();
        Persons.data=poissrnd(lambda);
      state Wait
      (default) -> Hour_11.min_30.IDLE : {dt=0;}
      Hour_11.min_30.Wait -> Hour_11.min_30.IDLE : after(dt,sec){send(Persons)}
      Hour_11.min_30.IDLE -> Hour_11.min_30.Wait
    (default) -> Hour_11.min_0
    Hour_11.min_0 -> Hour_11.min_15 : after(60*15,sec)
    Hour_11.min_30 -> Hour_11.min_45 : after(60*15,sec)
    Hour_11.min_15 -> Hour_11.min_30 : after(60*15,sec)
  state Hour_12
    state min_0
      state IDLE
        entry:
        lambda = 4;
        dt =60* rand();
        Persons.data=poissrnd(lambda);
      state Wait
      (default) -> Hour_12.min_0.IDLE
      Hour_12.min_0.Wait -> Hour_12.min_0.IDLE : after(dt,sec){send(Persons)}
      Hour_12.min_0.IDLE -> Hour_12.min_0.Wait
    state min_45
      state IDLE
        entry:
        lambda = 4;
        dt =60* rand();
        Persons.data=poissrnd(lambda);
      state Wait
      (default) -> Hour_12.min_45.IDLE : {dt=0;}
      Hour_12.min_45.Wait -> Hour_12.min_45.IDLE : after(dt,sec){send(Persons)}
      Hour_12.min_45.IDLE -> Hour_12.min_45.Wait
    state min_15
      state IDLE
        entry:
        lambda = 4;
        dt =60* rand();
        Persons.data=poissrnd(lambda);
      state Wait
      (default) -> Hour_12.min_15.IDLE : {dt=0;}
      Hour_12.min_15.Wait -> Hour_12.min_15.IDLE : after(dt,sec){send(Persons)}
      Hour_12.min_15.IDLE -> Hour_12.min_15.Wait
    state min_30
      state IDLE
        entry:
        lambda = 4;
        dt =60* rand();
        Persons.data=poissrnd(lambda);
      state Wait
      (default) -> Hour_12.min_30.IDLE : {dt=0;}
      Hour_12.min_30.Wait -> Hour_12.min_30.IDLE : after(dt,sec){send(Persons)}
      Hour_12.min_30.IDLE -> Hour_12.min_30.Wait
    (default) -> Hour_12.min_0
    Hour_12.min_0 -> Hour_12.min_15 : after(60*15,sec)
    Hour_12.min_30 -> Hour_12.min_45 : after(60*15,sec)
    Hour_12.min_15 -> Hour_12.min_30 : after(60*15,sec)
  Hour_24 -> Hour_1 : after(60*60,sec)
  Hour_23 -> Hour_24 : after(60*60,sec)
  Hour_22 -> Hour_23 : after(60*60,sec)
  (default) -> Hour_1 : {
      |  lambda=0;
      |  dt=0;
      |
      | }
  Hour_1 -> Hour_2 : after(60*60,sec)
  Hour_21 -> Hour_22 : after(60*60,sec)
  Hour_2 -> Hour_3 : after(60*60,sec)
  Hour_20 -> Hour_21 : after(60*60,sec)
  Hour_3 -> Hour_4 : after(60*60,sec)
  Hour_19 -> Hour_20 : after(60*60,sec)
  Hour_4 -> Hour_5 : after(60*60,sec)
  Hour_18 -> Hour_19 : after(60*60,sec)
  Hour_5 -> Hour_6 : after(60*60,sec)
  Hour_17 -> Hour_18 : after(60*60,sec)
  Hour_6 -> Hour_7 : after(60*60,sec)
  Hour_16 -> Hour_17 : after(60*60,sec)
  Hour_7 -> Hour_8 : after(60*60,sec)
  Hour_15 -> Hour_16 : after(60*60,sec)
  Hour_8 -> Hour_9 : after(60*60,sec)
  Hour_14 -> Hour_15 : after(60*60,sec)
  Hour_13 -> Hour_14 : after(60*60,sec)
  Hour_9 -> Hour_10 : after(60*60,sec)
  Hour_10 -> Hour_11 : after(60*60,sec)
  Hour_12 -> Hour_13 : after(60*60,sec)
  Hour_11 -> Hour_12 : after(60*60,sec)
  data: Persons output; dt local; lambda local
